simulink model "Pressure_I2C_BMP388_4"  (R2022b)
settings: Solver=FixedStepDiscrete  StartTime=0.0  StopTime=inf  RelTol=1e-3  EnableMultiTasking=on
InitFcn:
  | mbd_s32k_consistency_checks(bdroot(gcs));
model workspace (MAT data in the model file):
  mwTaskManagerKernelLatency = 1e-06
undefined symbols (not defined in the file): LQFP
libraries: mbd_s32k1xx_ec_toolbox x7, hdlsllib x1
settings Model: Creator=kamil  LastModifiedBy=kamil
settings SolverCC: PositivePriorityOrder=on
settings DataIOCC: ExternalInput=off  InitialState=off  SaveOutput=off  SignalLogging=off  SaveTime=off
settings OptimizationCC: DefaultParameterBehavior=Inlined  EnhancedBackFolding=on  PassReuseOutputArgsAs=Individual arguments  ZeroExternalMemoryAtStartup=off  ZeroInternalMemoryAtStartup=off  MaxStackSize=64  OptimizeBlockOrder=speed  DifferentSizesBufferReuse=on  OptimizationCustomize=off  EfficientTunableParamExpr=on
settings DebuggingCC: InheritedTsInSrcMsg=none  ParameterTunabilityLossMsg=error
settings HardwareCC: ProdBitPerPointer=32  ProdBitPerSizeT=32  ProdBitPerPtrDiffT=32  ProdLargestAtomicInteger=Long  ProdLargestAtomicFloat=Double  ProdWordSize=32  ProdHWDeviceType=ARM Compatible->ARM Cortex  HardwareBoardFeatureSet=SoCBlockset
settings ModelReferenceCC: PropagateSignalLabelsOutOfModel=off
settings SFSimCC: SimUserSources=bmp3.c  MATLABDynamicMemAlloc=off  CustomCodeUndefinedFunction=UseInterfaceOnly
settings SFSimCC: SimCustomHeaderCode=|
  | #include "bmp3.h"
  | #include "bmp3_defs.h"
settings RTWCC: Description=Model Based Design Toolbox S32K1xx Code Generation Target  SystemTargetFile=mbd_s32k.tlc  MakeCommand=mbd_s32k_make_rtw COPY_MDLREF_INCLUDES=0  TemplateMakefile=mbd_s32k.tmf  GenerateReport=on  LaunchReport=on
settings CodeAppCC: ForceParamTrailComments=on  IgnoreCustomStorageClasses=off  OperatorAnnotations=on  SimulinkDataObjDesc=on  SFDataObjDesc=on  InsertBlockDesc=on
settings STFCustomTargetCC: MultiwordLength=256  CombineOutputUpdateFcns=on  ERTCustomFileBanners=on  SupportContinuousTime=off  SupportNonInlinedSFcns=off  RemoveResetFunc=on  MATLABClassNameForMDSCustomization=Simulink.SoftwareTarget.ERTCustomization  SystemTargetFile=mbd_s32k.tlc
settings ERTTargetCC: ParMdlRefBuildCompliant=off  CompOptLevelCompliant=off  ConcurrentExecutionCompliant=off  ModelStepFunctionPrototypeControlCompliant=off  CPPClassGenCompliant=off  UseToolchainInfoCompliant=off  InlinedParameterPlacement=NonHierarchical  ERTCustomFileTemplate=example_file_process.tlc

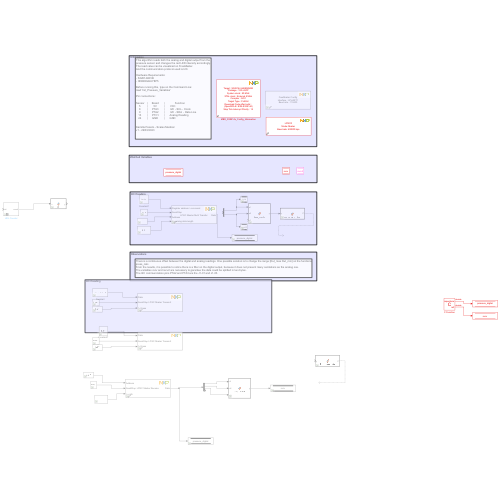
[thumbnail: Simulink's stored preview of the top-level diagram]
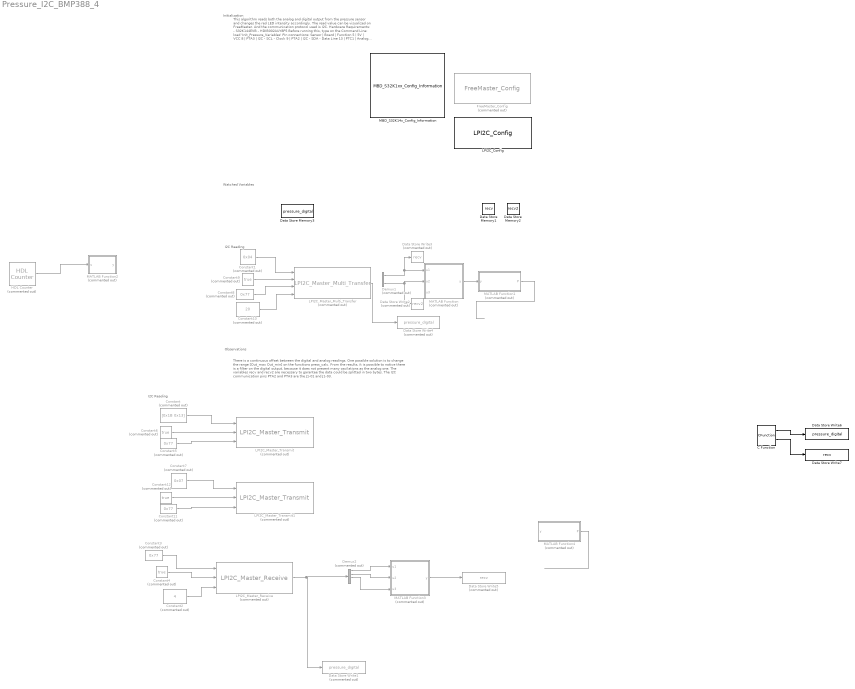
== system Pressure_I2C_BMP388_4 ==
  note: This algorithm reads both the analog and digital output from the
      | pressure sensor and changes the red LED intensity accordingly.
      | The read value can be visualized on FreeMaster.
      | And the communication protocol used is I2C.
      |
      | Hardware Requirements:
      | - S32K144EVB
      | - HDIB002AUY8P5
      |
      | Before running this, type on the Command Line:
      | load 'Init_Pressure_Variables'
      |
      | Pin connections:
      |
      | Sensor    |     Board       |              Function
      |     5         |        5V          |       VCC
      |     8         |      PTA3        |       I2C - SCL - Clock
      |     9         |      PTA2        |       I2C - SDA  - Data Line
      |    13        |      PTC1       |       Analog Reading
      |    24        |      GND        |       GND
      |
      |
      | Kamilla Peixoto - Scaleo Medical
      | v1 - 29/03/2023
  note: I2C Reading
  note: Watched Variables
  note: Initialization
  note: Observations
  note: There is a continuous offset between the digital and analog readings. One possible solution is to change the range [Out_max Out_min] on the functions
      | press_calc.
      | From the results, it is possible to notice there is a filter on the digital output, because it does not present many oscilations as the analog one.
      | The variables recv and recv2 are necessary to garantee the data could be splitted in two bytes.
      | The I2C communication pins PTA2 and PTA3 are the J1-01 and J1-03.
  note: I2C Reading
  C Function : CFunction  OutputCode=|
      | struct bmp3_data data_sens;
      |  struct bmp3_dev the_sensor;
      |  double temp;
      |   
      |   uint8_t sensor_comp = 0;
      |   sensor_comp |= BMP3_TEMP;
      |  
      |   rslt = bmp3_get_sensor_data(0, &data_sens, &the_sensor);
      |  
      |   temp = data_sens.temperature;
      |   
      |   temperature = temp;
  Constant : Constant  Commented=on  Value=[0x1B 0x13]  VectorParams1D=off  SampleTime=-1
  Constant1 : Constant  Commented=on  Value=0x04  VectorParams1D=off  SampleTime=-1
  Constant10 : Constant  Commented=on  Value=20  OutDataTypeStr=uint32
  Constant{3,5,8,11} (4 alike) : Constant  Commented=on  Value=0x77  OutDataTypeStr=uint16
  Constant{4,6,9,12} (4 alike) : Constant  Commented=on  Value=true  OutDataTypeStr=boolean
  Constant2 : Constant  Commented=on  Value=4  OutDataTypeStr=uint32
  Constant7 : Constant  Commented=on  Value=0x07  VectorParams1D=off  SampleTime=-1
  Data Store Memory1 : DataStoreMemory  DataStoreName=recv  ReadBeforeWriteMsg=warning  WriteAfterWriteMsg=warning  WriteAfterReadMsg=warning  ShowAdditionalParam=off  StateMustResolveToSignalObject=on
  Data Store Memory2 : DataStoreMemory  DataStoreName=recv2  ReadBeforeWriteMsg=warning  WriteAfterWriteMsg=warning  WriteAfterReadMsg=warning  ShowAdditionalParam=off  OutDataTypeStr=uint8
  Data Store Memory3 : DataStoreMemory  DataStoreName=pressure_digital  WriteAfterWriteMsg=warning  InitialValue=zeros(1, 1)  ShowAdditionalParam=off  StateMustResolveToSignalObject=on
  Data Store Write1 : DataStoreWrite  Commented=on  DataStoreName=pressure_digital  IndexOptions=Index vector (dialog)  Indices=1  OutputSizes=1
  Data Store Write2 : DataStoreWrite  Commented=on  DataStoreName=recv2  IndexOptions=Index vector (dialog)  Indices=1  OutputSizes=1
  Data Store Write3 : DataStoreWrite  Commented=on  DataStoreName=recv  IndexOptions=Index vector (dialog)  Indices=1  OutputSizes=1
  Data Store Write4 : DataStoreWrite  Commented=on  DataStoreName=pressure_digital  IndexOptions=Index vector (dialog)  Indices=1  OutputSizes=1
  Data Store Write5 : DataStoreWrite  Commented=on  DataStoreName=recv  IndexOptions=Index vector (dialog)  Indices=1  OutputSizes=1
  Data Store Write6 : DataStoreWrite  DataStoreName=pressure_digital  IndexOptions=Index vector (dialog)  Indices=1  OutputSizes=1
  Data Store Write7 : DataStoreWrite  DataStoreName=recv  IndexOptions=Index vector (dialog)  Indices=1  OutputSizes=1
  Demux1 : Demux  Commented=on  Outputs=2
  Demux2 : Demux  Commented=on
  FreeMaster_Config : mbd_s32k1xx_ec_toolbox/Utility Blocks/FreeMaster_Config  Commented=on  interface=LPUART1  baudrate=115200  rxd=PTC6: [LPUART1_RX | Receive]  txd=PTC7: [LPUART1_TX | Transmit]  mode=Poll-driven  isr_prio=15  show_adv_opts=on  use_scope=on  max_scope_vars=8  use_recorder=on  max_rec_vars=8  rec_buff_size=1024  rec_timebase=0 seconds  comm_buffer_size_auto=on  comm_buffer_size=255  comm_rqueue_size_default=on  comm_rqueue_size=32
  HDL Counter : hdlsllib/Sources/HDL Counter  Commented=on  CountType=Count limited  CountInit=0  CountStep=1  CountMax=25  CountFromType=Initial value  CountFrom=0  CountResetPort=on  CountLoadPort=off  CountEnbPort=off  CountDirPort=off  CountHitOutputPort=off  CountDataType=Unsigned  CountWordLen=8  CountFracLen=0  CountSampTime=1
  LPI2C_Config : mbd_s32k1xx_ec_toolbox/Communication Blocks/I2C Blocks/LPI2C_Config  Priority=1  instance=0  mode=Master  opmode=Standard (up to 100 kbit/s)  bdr=400000  addr=1  is10bitaddr=off  sda=PTA2: [LPI2C0_SDA | LPI2C Data I/O]  scl=PTA3: [LPI2C0_SCL | LPI2C Clock I/O]
  LPI2C_Master_Multi_Transfer : mbd_s32k1xx_ec_toolbox/Communication Blocks/I2C Blocks/LPI2C_Master_Multi_Transfer  Priority=3  Commented=on  instance=0  xfermode=Blocking  Timeout=50  delay_between_transfers=50  is10bit=off
  LPI2C_Master_Receive : mbd_s32k1xx_ec_toolbox/Communication Blocks/I2C Blocks/LPI2C_Master_Receive  Priority=4  Commented=on  instance=0  xfermode=Blocking  Timeout=50  is10bit=off
  LPI2C_Master_Transmit : mbd_s32k1xx_ec_toolbox/Communication Blocks/I2C Blocks/LPI2C_Master_Transmit  Priority=2  Commented=on  instance=0  xfermode=Blocking  Timeout=50  is10bit=off
  LPI2C_Master_Transmit1 : mbd_s32k1xx_ec_toolbox/Communication Blocks/I2C Blocks/LPI2C_Master_Transmit  Priority=3  Commented=on  instance=0  xfermode=Blocking  Timeout=50  is10bit=off
  MATLAB Function : MATLAB Function  Commented=on  TreatAsAtomicUnit=on
  MATLAB Function1 : MATLAB Function  Commented=on  TreatAsAtomicUnit=on
  MATLAB Function2 : MATLAB Function  Commented=on  TreatAsAtomicUnit=on
  MATLAB Function3 : MATLAB Function  Commented=on  TreatAsAtomicUnit=on
  MATLAB Function4 : MATLAB Function  Commented=on  TreatAsAtomicUnit=on
  MBD_S32K14x_Config_Information : mbd_s32k1xx_ec_toolbox/MBD_S32K1xx_Config_Information  Priority=0  mbdt_ver=0  disp_str=|  config_params=[]  mcu_target_name=S32K144  mcu_target_package=100-LQFP  mcu_target_sram_size=64KB  mcu_system_clock_freq=80  mcu_xtal_freq=External 8  mcu_steptick_timer=LPIT Channel 0  mcu_steptick_prio=15  ds_import_enable=on  target_compiler=GCC  target_memory=FLASH  gcc_target_compile_opts=-mcpu=cortex-m4 -mthumb -mfloat-abi=hard -mfpu=fpv4-sp-d16 -O1 -g -gstrict-dwarf  gcc_target_assemble_opts=-mcpu=cortex-m4 -mthumb -mfloat-abi=hard -mfpu=fpv4-sp-d16 -g  gcc_target_link_opts=-mcpu=cortex-m4 -mthumb -mfloat-abi=hard -mfpu=fpv4-sp-d16  gcc_target_default_lcf=on  gcc_target_user_lcf=S32K148_192_flash.ld  ghs_target_compile_opts=-cpu=cortexm4f -thumb -DARM_MATH_CM4 -fpu=vfpv4_d16 -fsingle -Ogeneral -Wundef -Wimplicit-int -Wshadow -Wtrigraphs --no_commons --gnu_asm -gnu99 -gdwarf-2 -G  ghs_target_assemble_opts=-cpu=cortexm4f -fpu=vfpv4_d16  ghs_target_link_opts=-cpu=cortexm4f -thumb -fpu=vfpv4_d16  ghs_target_default_lcf=off  ghs_target_user_lcf=S32K148_192_flash.ld  iar_target_compile_opts=--cpu=Cortex-M4F --thumb --fpu=VFPv4_sp -Ol -e --debug --dlib_config normal  iar_target_assemble_opts=--cpu Cortex-M4F --thumb --fpu VFPv4_sp  iar_target_link_opts=--no_exceptions --vfe --inline  iar_target_default_lcf=off  iar_target_user_lcf=S32K148_192_flash.icf  pil_download_enable=off  rbl_download_enable=on  rbl_start_delay=5000000  rbl_download_interface=OpenSDA  rbl_restart_request=off  rbl_com_port=Custom  rbl_com_port_custom=COM1  pil_download_rate=57600  pil_opensda_drive=E: EVB-S32K144  pil_opensda_drive_custom=D  pil_uart_instance=1  pil_uart_rx=PTC6: [LPUART1_RX | Receive]  pil_uart_tx=PTC7: [LPUART1_TX | Transmit]  FTM_PWM_PcrCheckEnDis=on  FTM_Input_Edge_Inputs_PcrCheckEnDis=on  FTM_Dual_Edge_Inputs_PcrCheckEnDis=on  FTM_Quadrature_Inputs_PcrCheckEnDis=on  FTM_Hall_Sensor_Inputs_PcrCheckEnDis=on  LPTMR_PcrCheckEnDis=on  PIT_PcrCheckEnDis=on  RTC_PcrCheckEnDis=on  FlexCAN_PcrCheckEnDis=on  LIN_PcrCheckEnDis=on  FlexIO_PcrCheckEnDis=on  LPI2C_PcrCheckEnDis=on  LPSPI_PcrCheckEnDis=on  LPUART_PcrCheckEnDis=on  CMP_PcrCheckEnDis=on  GPIO_OutputPcrCheckEnDis=on  GPIO_InputPcrCheckEnDis=on  SBC_PcrCheckEnDis=on  BMS_PcrCheckEnDis=on  AMMCLIB_PcrCheckEnDis=on  FM_PcrCheckEnDis=on  Profile_PcrCheckEnDis=on  ConfigParams_PcrCheckEnDis=on  ModelRef_PcrCheckEnDis=on  PDB0_PcrCheckEnDis=on  CSEc_PcrCheckEnDis=on  eDMA_PcrCheckEnDis=on  FLASH_PcrCheckEnDis=on  ADC_PcrCheckEnDis=on  WDOG_PcrCheckEnDis=on
      | Target : S32K144-64KB_SRAM
      | Package : 100-pin
      | System clock : 80 MHz
      | XTAL clock : External 8 MHz
      | Compiler : GCC
      | Target Type : FLASH
      | Download Code after build : (OpenSDA: E)
      | Step Tick Interrupt Priority : 15
  wires:
  MATLAB Function1/1(P) -> ?
  MATLAB Function/1(y) -> MATLAB Function1/1(y)
  Demux1/1 -> MATLAB Function/1(u1), Data Store Write3/1
  Constant10/1 -> LPI2C_Master_Multi_Transfer/4
  Demux1/2 -> Data Store Write2/1, MATLAB Function/2(u2)
  Constant9/1 -> LPI2C_Master_Multi_Transfer/2
  Constant8/1 -> LPI2C_Master_Multi_Transfer/3
  LPI2C_Master_Multi_Transfer/1 -> Data Store Write4/1
  LPI2C_Master_Receive/1 -> Demux2/1, Data Store Write1/1
  Constant4/1 -> LPI2C_Master_Receive/2
  Constant3/1 -> LPI2C_Master_Receive/1
  Constant2/1 -> LPI2C_Master_Receive/3
  HDL Counter/1 -> MATLAB Function2/1(u)
  Constant/1 -> LPI2C_Master_Transmit/1
  Constant5/1 -> LPI2C_Master_Transmit/3
  Constant6/1 -> LPI2C_Master_Transmit/2
  Constant1/1 -> LPI2C_Master_Multi_Transfer/1
  Constant7/1 -> LPI2C_Master_Transmit1/1
  Constant11/1 -> LPI2C_Master_Transmit1/3
  Constant12/1 -> LPI2C_Master_Transmit1/2
  MATLAB Function4/1(P) -> ?
  MATLAB Function3/1(y) -> Data Store Write5/1
  Demux2/1 -> MATLAB Function3/1(u1)
  Demux2/2 -> MATLAB Function3/2(u2)
  Demux2/3 -> MATLAB Function3/3(u3)
  C Function/1 -> Data Store Write6/1
  C Function/2 -> Data Store Write7/1

== matlab function Pressure_I2C_BMP388_4/MATLAB Function1 ==
  data: y input; P output
function P = press_calc_dig (y)
% Calculate the corresponding pressure based on the digital reading


%Pressure range
Pmax = 2000; %mbar
Pmin = 0;

%Digital range
Out_max_d = 29490;
Out_min_d = 3277;

S = (Out_max_d - Out_min_d)/(Pmax-Pmin);
P = (y - Out_min_d)/S + Pmin;

== matlab function Pressure_I2C_BMP388_4/MATLAB Function ==
  data: u1 input; y output; u2 input; u3 input
function y  = data_mask(u1, u2, u3)


u = [u1 u2 u3];

u_bin_mat = int2bit(u, 8);
u_bin_vec = (reshape(u_bin_mat, 1, []))';

y= bit2int(u_bin_vec, 24);

== matlab function Pressure_I2C_BMP388_4/MATLAB Function2 ==
  data: u input; y output
function y = fcn(u)
y = 0x1B;

if (u>1)
    y = 0x03;
end

== matlab function Pressure_I2C_BMP388_4/MATLAB Function3 ==
  data: u1 input; y output; u2 input; u3 input
function y  = data_mask(u1, u2, u3)


u = [u1 u2 u3];

u_bin_mat = int2bit(u, 8);
u_bin_vec = (reshape(u_bin_mat, 1, []))';

y= bit2int(u_bin_vec, 24);

== matlab function Pressure_I2C_BMP388_4/MATLAB Function4 ==
  data: y input; P output
function P = temp_calc_dig (y)
% Calculate the corresponding pressure based on the digital reading


%Pressure range
Tmax = 2000; %mbar
Tmin = 0;

%Digital range
Out_max_d = 29490;
Out_min_d = 3277;

S = (Out_max_d - Out_min_d)/(Tmax-Tmin);
P = (y - Out_min_d)/S + Tmin;
